simulink model "Control_PID_sim"  (R2021a)
settings: Solver=VariableStepAuto  StartTime=0.0  StopTime=runTime  MaxStep=1e-5  RelTol=1e-7  AbsTol=1e-7
undefined symbols (not defined in the file or in its folder): Cd, Crd, delay, K, P, Pd, ts, Ts
settings Model: Creator=Fran  LastModifiedBy=Francisco

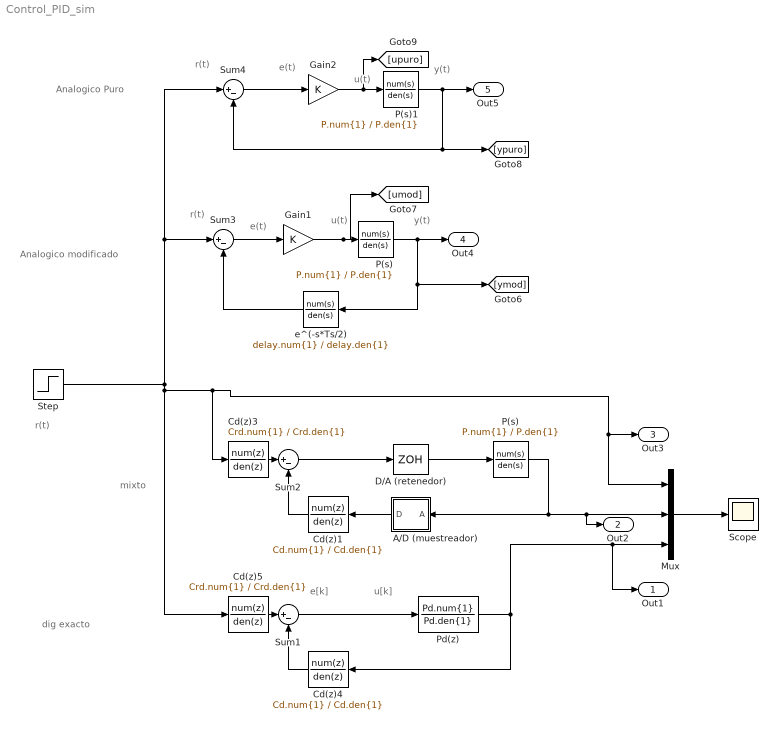
== system Control_PID_sim ==
  note: mixto
  note: dig exacto
  note: r(t)
  note: u[k]
  note: e[k]
  note: Analogico modificado
  note: r(t)
  note: u(t)
  note: y(t)
  note: Analogico Puro
  note: r(t)
  note: e(t)
  note: u(t)
  note: y(t)
  note: e(t)
  A/D (muestreador) : Subsystem
  Cd(z)1 : DiscreteTransferFcn  Numerator=Cd.num{1}  Denominator=Cd.den{1}  SampleTime=ts
  Cd(z)3 : DiscreteTransferFcn  Numerator=Crd.num{1}  Denominator=Crd.den{1}  SampleTime=ts
  Cd(z)4 : DiscreteTransferFcn  Numerator=Cd.num{1}  Denominator=Cd.den{1}  SampleTime=ts
  Cd(z)5 : DiscreteTransferFcn  Numerator=Crd.num{1}  Denominator=Crd.den{1}  SampleTime=ts
  D/A (retenedor) : ZeroOrderHold  SampleTime=ts
  Gain1 : Gain  Gain=K
  Gain2 : Gain  Gain=K
  Mux : Mux  Inputs=3
  P(s) : TransferFcn  Numerator=P.num{1}  Denominator=P.den{1}
  "P(s) " : TransferFcn  Numerator=P.num{1}  Denominator=P.den{1}
  P(s)1 : TransferFcn  Numerator=P.num{1}  Denominator=P.den{1}
  Pd(z) : DiscreteTransferFcn  Numerator=Pd.num{1}  Denominator=Pd.den{1}  SampleTime=Ts
  Scope : Scope
  Step : Step  SampleTime=0
  Sum{1..4} (4 alike) : Sum  Inputs=|+-
  e^(-s*Ts/2) : TransferFcn  Numerator=delay.num{1}  Denominator=delay.den{1}
  Out1 : Outport  SignalName=Dig Exacto
  Out2 : Outport  Port=2  SignalName=Mixto
  Out3 : Outport  Port=3  SignalName=R
  Out4 : Outport  Port=4  SignalName=An_Mod
  Out5 : Outport  Port=5  SignalName=An_Puro
  wires:
  "P(s) "/1 -> Out2/1, Mux/2, A/D (muestreador)/1(A)
  D/A (retenedor)/1 -> "P(s) "/1
  Sum2/1 -> D/A (retenedor)/1
  Mux/1 -> Scope/1
  A/D (muestreador)/1(D) -> Cd(z)1/1
  Cd(z)1/1 -> Sum2/2
  Cd(z)3/1 -> Sum2/1
  Cd(z)4/1 -> Sum1/2
  Pd(z)/1 -> Cd(z)4/1, Out1/1, Mux/3
  Cd(z)5/1 -> Sum1/1
  Sum1/1 -> Pd(z)/1
  P(s)1/1 -> [ypuro], Sum4/2, Out5/1
  Sum4/1 -> Gain2/1
  Sum3/1 -> Gain1/1
  Gain2/1 -> [upuro], P(s)1/1
  P(s)/1 -> [ymod], e^(-s*Ts/2)/1, Out4/1
  Gain1/1 -> [umod], P(s)/1
  e^(-s*Ts/2)/1 -> Sum3/2
  Step/1 -> Cd(z)5/1, Cd(z)3/1, Out3/1, Mux/1, Sum4/1, Sum3/1

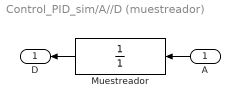
== system Control_PID_sim/A//D (muestreador) ==
  A : Inport
  Muestreador : DiscreteTransferFcn  Numerator=1  Denominator=1  SampleTime=ts
  D : Outport
  wires:
  A/1 -> Muestreador/1
  Muestreador/1 -> D/1
